simulink model "test_total_system"  (R2025b)
settings: Solver=FixedStepAuto  StartTime=0.0  StopTime=10.0  FixedStep=Ts  RelTol=1e-3
settings Model: TunableVars=J_AD,J_ICE,M_AD_nom,P_ballast_nom,P_oil_max,P_oil_min,T_AD_max,T_amb,T_ballast_max,T_cool_max,a_const,ad_fun_acceleration,b_const,k_heat,k_loss,k_loss0,k_rad_AD,k_rad_ballast,k_radiator,omega_ICE_max_prir,omega_ICE_max_run,tau,tau_AD_base,tau_ballast,tau_cool  TunableVarsStorageClass=Auto,Auto,Auto,Auto,Auto,Auto,Auto,Auto,Auto,Auto,Auto,Auto,Auto,Auto,Auto,Auto,Auto,Auto,Auto,Auto,Auto,Auto,Auto,Auto,Auto  TunableVarsTypeQualifier=,,,,,,,,,,,,,,,,,,,,,,,,  Creator=user  LastModifiedBy=user
settings OptimizationCC: DefaultParameterBehavior=Inlined  UseDivisionForNetSlopeComputation=on  GainParamInheritBuiltInType=on  UseFloatMulNetSlope=on  StrengthReduction=on  PassReuseOutputArgsAs=Individual arguments  ZeroExternalMemoryAtStartup=off  ZeroInternalMemoryAtStartup=off  NoFixptDivByZeroProtection=on  EfficientFloat2IntCast=on  OptimizeBlockOrder=speed  OptimizationPriority=Speed  OptimizationCustomize=off  MultiThreadedLoops=on  AutoScheduleForLoops=on  EfficientTunableParamExpr=on
settings DebuggingCC: ParameterTunabilityLossMsg=error
settings HardwareCC: ProdBitPerLong=64.0  ProdLongLongMode=on  ProdHWDeviceType=Intel->x86-64 (Linux 64)
settings SFSimCC: MATLABDynamicMemAlloc=off  SimTargetLang=C++  SimDLTargetLibrary=mkl-dnn
settings RTWCC: SystemTargetFile=ert.tlc  GenCodeOnly=on  TemplateMakefile=ert_default_tmf  GenerateReport=on  BuildConfiguration=Faster Runs  LaunchReport=on  TargetLang=C++  Description=Embedded Coder
settings CodeAppCC: ForceParamTrailComments=on  IgnoreCustomStorageClasses=off  OperatorAnnotations=on  SimulinkDataObjDesc=on  SFDataObjDesc=on  CustomSymbolStrGlobalVar=rt$N$M  CustomSymbolStrType=$N$M  CustomSymbolStrFcn=$N$M$F  CustomSymbolStrMacro=$N$M  InsertBlockDesc=on
settings ERTTargetCC: InlinedParameterPlacement=Hierarchical  RootIOFormat=Structure reference  ERTCustomFileTemplate=example_file_process.tlc  TargetLangStandard=C++17 (ISO)  GenerateSampleERTMain=on  CodeInterfacePackaging=C++ class  SubcomponentCodeInterfacePackaging=C++ class  SupportContinuousTime=on

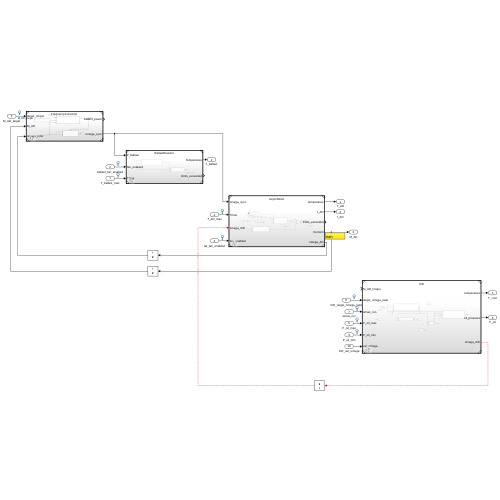
[thumbnail: Simulink's stored preview of the top-level diagram]
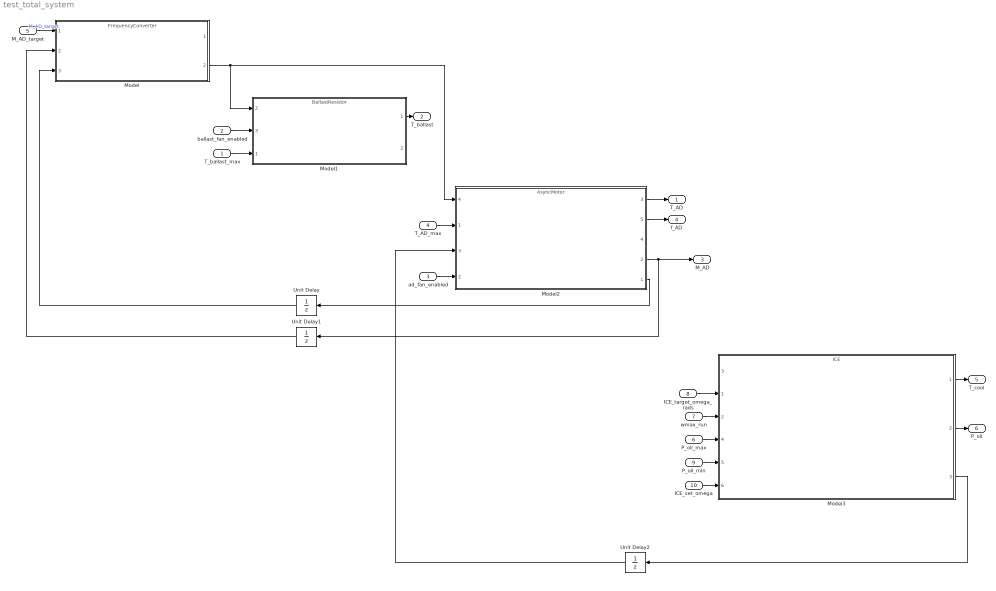
== system test_total_system ==
  T_ballast_max : Inport
  ballast_fan_enabled : Inport  Port=2
  ad_fan_enabled : Inport  Port=3
  T_AD_max : Inport  Port=4
  M_AD_target : Inport  Port=5
  P_oil_max : Inport  Port=6
  wmax_run : Inport  Port=7
  ICE_target_omega_rads : Inport  Port=8
  P_oil_min : Inport  Port=9
  ICE_set_omega : Inport  Port=10
  Model : ModelReference  ModelNameDialog=FrequencyConverter.slx  SimulationMode=Normal  ModelReferenceVersion=1.231
  Model1 : ModelReference  ModelNameDialog=BallastResistor.slx  SimulationMode=Normal  ModelReferenceVersion=1.226
      settings: PortSchema="{\"entries\":[{\"content\":{\"sides\":[{\"content\":{\"connectorIds\":[\"In2\",\"In3\",\"In1\"]},\"type\":\"ConnectorPlacement.EquallySpacedRectSide\",\"uuid\":\"7f109583-06ea-4128-9ee5-b1f60cf269dc\"},{\"content\":{\"connectorIds\":[\"Out1\",\"Out2\"],\"side\":\"RIGHT\"},\"type\":\"ConnectorPlacement.EquallySpacedRectSide\",\"uuid\":\"3ed18453-e43c-4600-8919-fb5fb0e1ce83\"},{\"content\":{\"side\":\"TOP\"},\"type\":\"ConnectorPlacement.EquallySpacedRectSide\",\"uuid\":\"5bef5430-3b3c-4fa1-bb01-31f9fd9d9302\"}]},\"type\":\"ConnectorPlacement.EquallySpacedConnector\",\"uuid\":\"126d711d-4c62-4e17-b781-2a3b986b6ad3\"}],\"packageUris\":[\"http://schema.mathworks.com/mf0/Connector/R2020b\"],\"version\":\"1.0\"}"
  Model2 : ModelReference  ModelNameDialog=AsyncMotor.slx  SimulationMode=Normal  ModelReferenceVersion=1.277
      settings: PortSchema="{\"entries\":[{\"content\":{\"sides\":[{\"content\":{\"connectorIds\":[\"In4\",\"In1\",\"In3\",\"In2\"]},\"type\":\"ConnectorPlacement.EquallySpacedRectSide\",\"uuid\":\"f6c3bdce-8207-4ba4-a070-5c73a9d0b9d5\"},{\"content\":{\"connectorIds\":[\"Out3\",\"Out5\",\"Out4\",\"Out2\",\"Out1\"],\"side\":\"RIGHT\"},\"type\":\"ConnectorPlacement.EquallySpacedRectSide\",\"uuid\":\"e5e1f6d3-cef5-4133-bdae-1a7d1828e713\"},{\"content\":{\"side\":\"TOP\"},\"type\":\"ConnectorPlacement.EquallySpacedRectSide\",\"uuid\":\"e9dee3fa-101b-4d4f-919d-f842b136fb42\"}]},\"type\":\"ConnectorPlacement.EquallySpacedConnector\",\"uuid\":\"28a5e948-9d87-40f7-8783-929a5f74df30\"}],\"packageUris\":[\"http://schema.mathworks.com/mf0/Connector/R2020b\"],\"version\":\"1.0\"}"
  Model3 : ModelReference  ModelNameDialog=ICE.slx  SimulationMode=Normal  ModelReferenceVersion=1.408
      settings: PortSchema="{\"entries\":[{\"content\":{\"sides\":[{\"content\":{\"connectorIds\":[\"In3\",\"In1\",\"In2\",\"In4\",\"In5\",\"In6\"]},\"type\":\"ConnectorPlacement.EquallySpacedRectSide\",\"uuid\":\"03a90139-1e88-4267-b314-cfb62ce18d1a\"},{\"content\":{\"connectorIds\":[\"Out1\",\"Out2\",\"Out3\"],\"side\":\"RIGHT\"},\"type\":\"ConnectorPlacement.EquallySpacedRectSide\",\"uuid\":\"8d42cf4f-92cc-4bcf-ab8f-3d0b14eeba6d\"},{\"content\":{\"side\":\"TOP\"},\"type\":\"ConnectorPlacement.EquallySpacedRectSide\",\"uuid\":\"ec99585d-049d-4d71-a81c-ffb7baa0e97b\"}]},\"type\":\"ConnectorPlacement.EquallySpacedConnector\",\"uuid\":\"e88772a1-3eed-4319-bd37-78f8632c8d7a\"}],\"packageUris\":[\"http://schema.mathworks.com/mf0/Connector/R2020b\"],\"version\":\"1.0\"}"
  Unit Delay : UnitDelay  SampleTime=-1  HasFrameUpgradeWarning=on
  Unit Delay1 : UnitDelay  SampleTime=-1  HasFrameUpgradeWarning=on
  Unit Delay2 : UnitDelay  SampleTime=-1  HasFrameUpgradeWarning=on
  T_AD : Outport
  T_ballast : Outport  Port=2
  M_AD : Outport  Port=3
  f_AD : Outport  Port=4
  T_cool : Outport  Port=5
  P_oil : Outport  Port=6
  wires:
  ad_fan_enabled/1 -> Model2/2
  T_AD_max/1 -> Model2/1
  Model2/3 -> T_AD/1
  Model1/1 -> T_ballast/1
  Model2/2 -> M_AD/1, Unit Delay1/1
  Model2/5 -> f_AD/1
  Model/2 -> Model1/2, Model2/4
  ballast_fan_enabled/1 -> Model1/3
  T_ballast_max/1 -> Model1/1
  Model2/1 -> Unit Delay/1
  Unit Delay/1 -> Model/3
  Unit Delay1/1 -> Model/2
  M_AD_target/1 -> Model/1  "M_AD_target"
  Model3/3 -> Unit Delay2/1
  Model3/1 -> T_cool/1
  Model3/2 -> P_oil/1
  P_oil_max/1 -> Model3/4
  wmax_run/1 -> Model3/2
  Unit Delay2/1 -> Model2/3
  ICE_target_omega_rads/1 -> Model3/1
  P_oil_min/1 -> Model3/5
  ICE_set_omega/1 -> Model3/6
